simulink model "Test"  (R2018b)
settings: Solver=VariableStepAuto  StartTime=0.0  StopTime=10.0  RelTol=1e-3
undefined symbols (not defined in the file or in its folder): ExpectedOutputs, Inputs, sigbuilder_block, TestCase, TestInps, TestIters
libraries: fillib x3, library x2
(part 7 of 7)

== stateflow chart Test/Test Assessment Block2 ==
  settings: stateMachineType=SIMPLIFIED_MACHINE
  state Run
    if TestCase == 1
    verify(task_done ==  0);
    verify(inst_ptr == 0);
    verify(task_error == 0);
    verify(latch_addr ==  0)
    verify(write == 0)
    verify(ctrl == 0)
    verify(abort == 0)
    verify(fb_select == 0);
    end
    settings: description=|
        | Verify if in Init state all the outputs are reset to 0.
        | The instruction pointer should be reset to 0 to point to the first instruction in the sequence.
  state step2
    if TestCase == 2
    verify(task_done ==  0);
    verify(inst_ptr == 0);
    verify(task_error == 0);
    verify(latch_addr ==  0)
    verify(write == 0)
    verify(ctrl == 0)
    verify(abort == 0)
    verify(fb_select == 42);
    end
    settings: description=|
        | Verify that with a trigger from global sequencer, the task execution is initiated.
        | The state transitions from INIT to FB_SELECT.
        | Verify that the function number register and start instruction pointer register are latched to the first instruction in the sequence.
  state step3
    if TestCase == 2
    verify(task_done ==  0);
    verify(inst_ptr == 1);
    verify(task_error == 0);
    verify(latch_addr ==  0)
    verify(write == 0)
    verify(ctrl == 0)
    verify(abort == 0)
    verify(fb_select == 42);
    end
    settings: description=Verify that the instruction pointer increments.
  state step4
    if TestCase == 3
    verify(task_done ==  0);
    verify(inst_ptr == 1);
    verify(task_error == 0);
    verify(latch_addr ==  1)
    verify(int32(addr) == 32)
    verify(write == 0)
    verify(ctrl == 0)
    verify(abort == 0)
    verify(fb_select == 42);
    end
    settings: description=|
        | Verify that the state switches to Fetch automatically.
        | Verify that the fetch address in the instruction sequence is latched on the addr output.
  state step5
    if TestCase == 3
    verify(task_done ==  0);
    verify(inst_ptr == 1);
    verify(task_error == 0);
    verify(latch_addr ==  0)
    verify(write == 0)
    verify(ctrl == 0)
    verify(abort == 0)
    verify(fb_select == 42);
    end
    settings: description=Verify that there is one cycle of wait state for data to be available to function blocks from task memories.
  state step6
    if TestCase == 3
    verify(task_done ==  0);
    verify(inst_ptr == 1);
    verify(task_error == 0);
    verify(latch_addr ==  0)
    verify(write == 0)
    verify(ctrl == 1)
    verify(abort == 0)
    verify(fb_select == 42);
    end
    settings: description=Verify that a ctrl pulse is sent to function blocks to begin execution.
  state step7
    if TestCase == 3
    verify(task_done ==  0);
    verify(inst_ptr == 1);
    verify(task_error == 0);
    verify(latch_addr ==  0)
    verify(write == 0)
    verify(ctrl == 0)
    verify(abort == 0)
    verify(fb_select == 42);
    end
  state step8
    if TestCase == 3
    verify(task_done ==  0);
    verify(inst_ptr == 2);
    verify(task_error == 0);
    verify(latch_addr ==  0)
    verify(write == 0)
    verify(ctrl == 0)
    verify(abort == 0)
    verify(fb_select == 42);
    end
    settings: description=Verify that the instruction pointer is incremented.
  state step9
    if TestCase == 4
    verify(task_done ==  0);
    verify(inst_ptr == 2);
    verify(task_error == 0);
    verify(latch_addr ==  1)
    verify(write == 0)
    verify(ctrl == 0)
    verify(abort == 0)
    verify(fb_select == 42);
    end
    settings: description=|
        | Verify that the state remains in Fetch if the super state (upper 4 bits of Error Code in status signal) has not changed but the Error code data bits 22 through 27 has been incremented once indicating a super state iteration.
        | Verify that the next fetch address in the instruction sequence is latched on to the addr output.
  state step10
    if TestCase == 4
    verify(task_done ==  0);
    verify(inst_ptr == 2);
    verify(task_error == 0);
    verify(latch_addr ==  0)
    verify(write == 0)
    verify(ctrl == 0)
    verify(abort == 0)
    verify(fb_select == 42);
    end
    settings: description=Verify that there is one cycle of wait state for data to be available to function blocks from task memories.
  state step11
    if TestCase == 4
    verify(task_done ==  0);
    verify(inst_ptr == 2);
    verify(task_error == 0);
    verify(latch_addr ==  0)
    verify(write == 0)
    verify(ctrl == 1)
    verify(abort == 0)
    verify(fb_select == 42);
    end
    settings: description=Verify that a ctrl pulse is sent to function blocks to begin execution.
  state step12
    if TestCase == 4
    verify(task_done ==  0);
    verify(inst_ptr == 2);
    verify(task_error == 0);
    verify(latch_addr ==  0)
    verify(write == 0)
    verify(ctrl == 0)
    verify(abort == 0)
    verify(fb_select == 42);
    end
  state step13
    if TestCase == 4
    verify(task_done ==  0);
    verify(inst_ptr == 2);
    verify(task_error == 0);
    verify(latch_addr ==  0)
    verify(write == 0)
    verify(ctrl == 0)
    verify(abort == 0)
    verify(fb_select == 42);
    end
  state step14
    if TestCase == 4
    verify(task_done ==  0);
    verify(inst_ptr == 3);
    verify(task_error == 0);
    verify(latch_addr ==  0)
    verify(write == 0)
    verify(ctrl == 0)
    verify(abort == 0)
    verify(fb_select == 42);
    end
    settings: description=Verify that the instruction pointer is incremented.
  state step15
    if TestCase == 5
    verify(task_done ==  0);
    verify(inst_ptr == 3);
    verify(task_error == 0);
    verify(latch_addr ==  1)
    verify(write == 0)
    verify(ctrl == 0)
    verify(abort == 0)
    verify(fb_select == 42);
    end
    settings: description=|
        | Verify that the state remains in Fetch if the super state (upper 4 bits of Error Code in status signal) has not changed but the Error code data bits 22 through 27 has been incremented once indicating a super state iteration.
        | Verify that the next fetch address in the instruction sequence is latched on to the addr output.
  state step16
    if TestCase == 5
    verify(task_done ==  0);
    verify(inst_ptr == 3);
    verify(task_error == 0);
    verify(latch_addr ==  0)
    verify(write == 0)
    verify(ctrl == 0)
    verify(abort == 0)
    verify(fb_select == 42);
    end
    settings: description=Verify that there is one cycle of wait state for data to be available to function blocks from task memories.
  state step17
    if TestCase == 5
    verify(task_done ==  0);
    verify(inst_ptr == 3);
    verify(task_error == 0);
    verify(latch_addr ==  0)
    verify(write == 0)
    verify(ctrl == 1)
    verify(abort == 0)
    verify(fb_select == 42);
    end
    settings: description=Verify that a ctrl pulse is sent to function blocks.
  state step18
    if TestCase == 5
    verify(task_done ==  0);
    verify(inst_ptr == 3);
    verify(task_error == 0);
    verify(latch_addr ==  0)
    verify(write == 0)
    verify(ctrl == 0)
    verify(abort == 0)
    verify(fb_select == 42);
    end
  state step19
    if TestCase == 5
    verify(task_done ==  0);
    verify(inst_ptr == 3);
    verify(task_error == 0);
    verify(latch_addr ==  0)
    verify(write == 0)
    verify(ctrl == 0)
    verify(abort == 0)
    verify(fb_select == 42);
    end
  state step20
    if TestCase == 5
    verify(task_done ==  0);
    verify(inst_ptr == 4);
    verify(task_error == 0);
    verify(latch_addr ==  0)
    verify(write == 0)
    verify(ctrl == 0)
    verify(abort == 0)
    verify(fb_select == 42);
    end
    settings: description=Verify that the instruction pointer is incremented.
  state step21
    if TestCase == 6
    verify(task_done ==  0);
    verify(inst_ptr == 4);
    verify(task_error == 0);
    verify(latch_addr ==  0)
    verify(write == 0)
    verify(ctrl == 1)
    verify(abort == 0)
    verify(fb_select == 42);
    end
    settings: description=|
        | Verify that the state changes to Execute if the super state (upper 4 bits of Error Code in status signal) has changed indicating next state.
        | Verify that a ctrl pulse is sent to the function blocks for execution.
  state step22
    if TestCase == 6
    verify(task_done ==  0);
    verify(inst_ptr == 4);
    verify(task_error == 0);
    verify(latch_addr ==  0)
    verify(write == 0)
    verify(ctrl == 0)
    verify(abort == 0)
    verify(fb_select == 42);
    end
  state step23
    if TestCase == 7
    verify(task_done ==  0);
    verify(inst_ptr == 4);
    verify(task_error == 0);
    verify(latch_addr ==  1);
    verify(write == 0)
    verify(ctrl == 0)
    verify(abort == 0)
    verify(fb_select == 42);
    end
    settings: description=|
        | Verify that the state changes to Write if the super state (upper 4 bits of Error Code in status signal) has changed indicating next state.
        | Verify that the output address in the instruction sequence is latched on to the addr output.
  state step24
    if TestCase == 7
    verify(task_done ==  0);
    verify(inst_ptr == 4);
    verify(task_error == 0);
    verify(latch_addr ==  0);
    verify(write == 0)
    verify(ctrl == 1)
    verify(abort == 0)
    verify(fb_select == 42);
    end
    settings: description=Verify that a ctrl pulse is sent to function blocks.
  state step25
    if TestCase == 8
    verify(task_done ==  0);
    verify(inst_ptr == 4);
    verify(task_error == 0);
    verify(latch_addr ==  0);
    verify(write == 0)
    verify(ctrl == 0)
    verify(abort == 0)
    verify(fb_select == 42);
    end
  state step26
    if TestCase == 8
    verify(task_done ==  0);
    verify(inst_ptr == 4);
    verify(task_error == 0);
    verify(latch_addr ==  0);
    verify(write == 1)
    verify(ctrl == 0)
    verify(abort == 0)
    verify(fb_select == 42);
    end
    settings: description=Verify that the write output is set high to allow the function block to write the result to the current address.
  state step27
    if TestCase == 8
    verify(task_done ==  0);
    verify(inst_ptr == 4);
    verify(task_error == 0);
    verify(latch_addr ==  0);
    verify(write == 0)
    verify(ctrl == 0)
    verify(abort == 0)
    verify(fb_select == 42);
    end
  state step28
    if TestCase == 8
    verify(task_done ==  0);
    verify(inst_ptr == 5);
    verify(task_error == 0);
    verify(latch_addr ==  0);
    verify(write == 0)
    verify(ctrl == 0)
    verify(abort == 0)
    verify(fb_select == 42);
    end
    settings: description=Verify that the instruction pointer is incremented.
  state step29
    if TestCase == 9
    verify(task_done ==  0);
    verify(inst_ptr == 5);
    verify(task_error == 0);
    verify(latch_addr ==  1);
    verify(write == 0)
    verify(ctrl == 0)
    verify(abort == 0)
    verify(fb_select == 42);
    end
    settings: description=|
        | Verify that the state remains in Write if the super state (upper 4 bits of Error Code in status signal) has not changed but the Error code data bits 22 through 27 has been incremented once indicating a super state iteration.
        | Verify that the 2nd output address in the instruction sequence is latched on to the addr output.
  state step30
    if TestCase == 9
    verify(task_done ==  0);
    verify(inst_ptr == 5);
    verify(task_error == 0);
    verify(latch_addr ==  0);
    verify(write == 0)
    verify(ctrl == 1)
    verify(abort == 0)
    verify(fb_select == 42);
    end
    settings: description=Verify that a ctrl pulse is sent to function blocks.
  state step31
    if TestCase == 9
    verify(task_done ==  0);
    verify(inst_ptr == 5);
    verify(task_error == 0);
    verify(latch_addr ==  0);
    verify(write == 0)
    verify(ctrl == 0)
    verify(abort == 0)
    verify(fb_select == 42);
    end
  state step32
    if TestCase == 9
    verify(task_done ==  0);
    verify(inst_ptr == 5);
    verify(task_error == 0);
    verify(latch_addr ==  0);
    verify(write == 1)
    verify(ctrl == 0)
    verify(abort == 0)
    verify(fb_select == 42);
    end
    settings: description=Verify that the write output is set high to allow the function block to write the result to the current address.
  state step33
    if TestCase == 9
    verify(task_done ==  0);
    verify(inst_ptr == 5);
    verify(task_error == 0);
    verify(latch_addr ==  0);
    verify(write == 0)
    verify(ctrl == 0)
    verify(abort == 0)
    verify(fb_select == 42);
    end
  state step34
    if TestCase == 9
    verify(task_done ==  0);
    verify(inst_ptr == 6);
    verify(task_error == 0);
    verify(latch_addr ==  0);
    verify(write == 0)
    verify(ctrl == 0)
    verify(abort == 0)
    verify(fb_select == 42);
    end
    settings: description=Verify that the instruction pointer is incremented.
  state step35
    if TestCase == 9
    verify(task_done ==  0);
    verify(inst_ptr == 6);
    verify(task_error == 0);
    verify(latch_addr ==  0);
    verify(write == 0)
    verify(ctrl == 1)
    verify(abort == 0)
    verify(fb_select == 42);
    end
    settings: description=|
        | Verify that the state changes to FB_DONE if the super state (upper 4 bits of Error Code in status signal) has changed indicating next state.
        | Verify that a ctrl pulse is sent to function blocks to progress its state.
        | Verify that an Error while in FB_Done state does not cause it the local sequencer to move to the ERROR state.
  state step36
    if TestCase == 9
    verify(task_done ==  0);
    verify(inst_ptr == 6);
    verify(task_error == 0);
    verify(latch_addr ==  0);
    verify(write == 0)
    verify(ctrl == 0)
    verify(abort == 0)
    verify(fb_select == 42);
    end
  state step37
    if TestCase == 10
    verify(task_done ==  0);
    verify(inst_ptr == 6);
    verify(task_error == 0);
    verify(latch_addr ==  0);
    verify(write == 0)
    verify(ctrl == 0)
    verify(abort == 0)
    verify(fb_select == 42);
    end
    settings: description=Verify that the state changes to FB_SELECT if the super state (upper 4 bits of Error Code in status signal) has changed indicating next state.
  state step38
    if TestCase == 10
    verify(task_done ==  0);
    verify(inst_ptr == 6);
    verify(task_error == 0);
    verify(latch_addr ==  0);
    verify(write == 0)
    verify(ctrl == 0)
    verify(abort == 0)
    verify(fb_select == 41);
    end
    settings: description=Verify that the function number register and start instruction pointer register are latched to the 2nd function block instruction in the sequence.
  state step39
    if TestCase == 10
    verify(task_done ==  0);
    verify(inst_ptr == 7);
    verify(task_error == 0);
    verify(latch_addr ==  0);
    verify(write == 0)
    verify(ctrl == 0)
    verify(abort == 0)
    verify(fb_select == 41);
    end
    settings: description=|
        | Verify that the instruction pointer is incremented.
        | Verify that an Error while in FB_SELECT state does not cause it the local sequencer to move to the ERROR state.
  state step40
    if TestCase == 11
    verify(task_done ==  0);
    verify(inst_ptr == 7);
    verify(task_error == 0);
    verify(latch_addr ==  1);
    verify(write == 0)
    verify(ctrl == 0)
    verify(abort == 0)
    verify(fb_select == 41);
    end
    settings: description=|
        | Verify that the state switches to Fetch automatically.
        | Verify that the fetch address in the instruction sequence is latched on the addr output.
  state step41
    if TestCase == 11
    verify(task_done ==  0);
    verify(inst_ptr == 7);
    verify(task_error == 0);
    verify(latch_addr == 0);
    verify(write == 0)
    verify(ctrl == 1)
    verify(abort == 0)
    verify(fb_select == 41);
    end
    settings: description=|
        | Verify that the state switches to ERROR if the Error signal in Status input is true.
        | Verify that a ctrl pulse is sent to function blocks.
        | Verify that abort and Task_Error output signals are set to false if the lower 22 bits of the Code in Status signal indicate a recoverable error.
  state step42
    if TestCase == 11
    verify(task_done ==  0);
    verify(inst_ptr == 7);
    verify(task_error == 0);
    verify(latch_addr == 0);
    verify(write == 0)
    verify(ctrl == 0)
    verify(abort == 0)
    verify(fb_select == 41);
    end
  state step43
    if TestCase == 12
    verify(task_done ==  0);
    verify(inst_ptr == 7);
    verify(task_error == 0);
    verify(latch_addr == 0);
    verify(write == 0)
    verify(ctrl == 0)
    verify(abort == 0)
    verify(fb_select == 41);
    end
    settings: description=|
        | If the lower 22 bits of the Code in Status signal indicate a recoverable error,
        | verify that the state changes from ERROR to FB_SELECT.
  state step44
    if TestCase == 12
    verify(task_done ==  0);
    verify(inst_ptr == 6);
    verify(task_error == 0);
    verify(latch_addr == 0);
    verify(write == 0)
    verify(ctrl == 0)
    verify(abort == 0)
    verify(fb_select == 41);
    end
    settings: description=With a recoverable error verify that the instruction pointer is loaded with the value stored in the start instruction pointer register.
  state step45
    if TestCase == 12
    verify(task_done ==  0);
    verify(inst_ptr == 7);
    verify(task_error == 0);
    verify(latch_addr == 0);
    verify(write == 0)
    verify(ctrl == 0)
    verify(abort == 0)
    verify(fb_select == 41);
    end
    settings: description=Verify that the instruction pointer is incremented.
  state step46
    if TestCase == 13
    verify(task_done ==  0);
    verify(inst_ptr == 7);
    verify(task_error == 0);
    verify(latch_addr == 1);
    verify(write == 0)
    verify(ctrl == 0)
    verify(abort == 0)
    verify(fb_select == 41);
    end
    settings: description=|
        | Verify that the state switches to Fetch automatically.
        | Verify that the fetch address in the instruction sequence is latched on the addr output.
        | Verify that there is one cycle of wait state for data to be available to function blocks from task memories.
        | Verify that in the next cycle a ctrl pulse is sent to function blocks to begin execution.
        | Verify that after 2 cycles the instruction pointer is incremented.
  state step47
    if TestCase == 13
    verify(task_done ==  0);
    verify(inst_ptr == 7);
    verify(task_error == 0);
    verify(latch_addr == 0);
    verify(write == 0)
    verify(ctrl == 0)
    verify(abort == 0)
    verify(fb_select == 41);
    end
  state step48
    if TestCase == 13
    verify(task_done ==  0);
    verify(inst_ptr == 7);
    verify(task_error == 0);
    verify(latch_addr == 0);
    verify(write == 0)
    verify(ctrl == 1)
    verify(abort == 0)
    verify(fb_select == 41);
    end
  state step49
    if TestCase == 13
    verify(task_done ==  0);
    verify(inst_ptr == 7);
    verify(task_error == 0);
    verify(latch_addr == 0);
    verify(write == 0)
    verify(ctrl == 0)
    verify(abort == 0)
    verify(fb_select == 41);
    end
  state step50
    if TestCase == 13
    verify(task_done ==  0);
    verify(inst_ptr ==8)
    verify(task_error == 0);
    verify(latch_addr == 0)
    verify(write == 0)
    verify(ctrl == 0)
    verify(abort == 0)
    verify(fb_select == 41);
    end
  state step51
    if (TestCase == 14)
    verify(task_done ==  0);
    verify(inst_ptr ==8)
    verify(task_error == 0);
    verify(latch_addr == 0)
    verify(write == 0)
    verify(ctrl == 1)
    verify(abort == 0)
    verify(fb_select == 41);
    end
    settings: description=|
        | Verify that the state changes to Execute if the super state (upper 4 bits of Error Code in status signal) has changed indicating next state.
        | Verify that a ctrl pulse is sent to the function blocks for execution.
  state step52
    if (TestCase == 14)
    verify(task_done ==  0);
    verify(inst_ptr == 8)
    verify(task_error == 1);
    verify(latch_addr == 0)
    verify(write == 0)
    verify(ctrl == 1)
    verify(abort == 1)
    verify(fb_select == 41);
    end
    settings: description=|
        | Verify that the state switches to ERROR if the Error signal in Status input is true.
        | If the lower 22 bits of the Code in Status signal indicate a non recoverable error, verify that a ctrl and abort signals are pulsed for one cycle.
        | Verify that the Task_Error output is set to true until the Trigger goes low.
  state step53
    if (TestCase == 14)
    verify(task_done ==  0);
    verify(inst_ptr == 8)
    verify(task_error == 1);
    verify(latch_addr == 0)
    verify(write == 0)
    verify(ctrl == 0)
    verify(abort == 0)
    verify(fb_select == 41);
    end
  state step54
    if (TestCase == 15)
    verify(task_done ==  0);
    verify(inst_ptr == 0)
    verify(task_error == 0);
    verify(latch_addr == 0)
    verify(write == 0)
    verify(ctrl == 0)
    verify(abort == 0)
    verify(fb_select == 0);
    end
    settings: description=|
        | Verify that the state transitions from ERROR state to INIT if the error is not recoverable and the trigger from the global sequencer is low.
        | Verify if in Init state all the outputs are reset to 0.
        | The instruction pointer should be reset to 0 to point to the first instruction in the sequence
  state step55
    if (TestCase == 16)
    verify(task_done ==  0);
    verify(inst_ptr == 0)
    verify(task_error == 0);
    verify(latch_addr == 0)
    verify(write == 0)
    verify(ctrl == 0)
    verify(abort == 0)
    verify(fb_select == 50);
    end
    settings: description=|
        | Verify that with a trigger from global sequencer, the task execution is initiated.
        | The state transitions from INIT to FB_SELECT.
        | Verify that the function number register and start instruction pointer register are latched to the first instruction in the sequence.
  state step_1
  state step56
    if TestCase == 16
    verify(task_done ==  0);
    verify(inst_ptr == 2)
    verify(task_error == 0);
    verify(latch_addr == 1)
    verify(write == 0)
    verify(ctrl == 0)
    verify(abort == 0)
    verify(fb_select == 50);
    end
    settings: description=Verify that the write state is entered.
  state step_57
    if TestCase == 16
    verify(task_done ==  0);
    verify(inst_ptr == 2)
    verify(task_error == 0);
    verify(latch_addr == 0)
    verify(write == 0)
    verify(ctrl == 1)
    verify(abort == 0)
    verify(fb_select == 50);
    end
    settings: description=Verify that Error state is entered from write state if error is detected.
  state step_58
    if TestCase == 16
    verify(task_done ==  0);
    verify(inst_ptr == 2)
    verify(task_error == 0);
    verify(latch_addr == 0)
    verify(write == 0)
    verify(ctrl == 0)
    verify(abort == 0)
    verify(fb_select == 50);
    end
  state step59
    if TestCase ==16
    verify(task_done ==  0);
    verify(inst_ptr == 0)
    verify(task_error == 0);
    verify(latch_addr == 0)
    verify(write == 0)
    verify(ctrl == 0)
    verify(abort == 0)
    verify(fb_select == 50);
    end
  state step60
  state step61
    if (TestCase == 17)
    verify(task_done ==  1);
    verify(inst_ptr == 3)
    verify(task_error == 0);
    verify(latch_addr == 0)
    verify(write == 0)
    verify(ctrl == 0)
    verify(abort == 0)
    verify(fb_select == 50);
    end
    settings: description=Verify that state moves to Task_Done from FB_Done state once function block signals a new state and EOF flag is the current instruction.
  state step63
    if (TestCase == 18)
    verify(task_done ==  0);
    verify(inst_ptr == 3)
    verify(task_error == 0);
    verify(latch_addr == 0)
    verify(write == 0)
    verify(ctrl == 0)
    verify(abort == 0)
    verify(fb_select == 50);
    end
    settings: description=Verify that the state moves from Task_Done to INIT state once Trigger goes low.
  state step64
    if (TestCase == 18)
    verify(task_done ==  0);
    verify(inst_ptr == 0)
    verify(task_error == 0);
    verify(latch_addr == 0)
    verify(write == 0)
    verify(ctrl == 0)
    verify(abort == 0)
    verify(fb_select == 0);
    end
  state step65
  state step66
    if ((TestCase == 19)||(TestCase == 20)||(TestCase == 21)||(TestCase == 22))
    verify(task_done ==  0);
    verify(inst_ptr == 1)
    verify(task_error == 1);
    verify(latch_addr == 0)
    verify(write == 0)
    verify(ctrl == 1)
    verify(abort == 1)
    verify(fb_select == 52);
    elseif((TestCase == 23)||(TestCase == 24)||(TestCase == 25)||(TestCase == 26)||(TestCase == 27)||(TestCase == 28) || (TestCase == 29) ||  (TestCase == 30))
    verify(task_done ==  0);
    verify(inst_ptr == 2)
    verify(task_error == 1);
    verify(latch_addr == 0)
    verify(write == 0)
    verify(ctrl == 1)
    verify(abort == 1)
    verify(fb_select == 52);
    elseif((TestCase == 31) || (TestCase == 32))
    verify(task_done ==  0);
    verify(inst_ptr == 3)
    verify(task_error == 1);
    verify(latch_addr == 0)
    verify(write == 0)
    verify(ctrl == 1)
    verify(abort == 1)
    verify(fb_select == 52);
    end
  state EndTest
  (default) -> Run
  Run -> (junction 371) [order 2] : [after(3,sec) && (TestCase == 1)
      | ]
  (junction 371) -> (junction 363)
  Run -> step2 [order 1] : [after(3,sec) && TestCase > 1
      | ]
  step2 -> step3 : [after(1,sec)
      | ]
  step3 -> (junction 363) [order 2] : [after(1,sec) && TestCase == 2
      | ]
  (junction 363) -> (junction 304)
  step3 -> step4 [order 1] : [after(1,sec) && TestCase > 2
      | ]
  step4 -> step5 : [after(1,sec)
      | ]
  step5 -> step6 : [after(1,sec)
      | ]
  step6 -> step7 : [after(1,sec)
      | ]
  step7 -> step8 : [after(2, sec)
      | ]
  step8 -> (junction 304) [order 2] : [after(1,sec) && TestCase == 3
      | ]
  (junction 304) -> (junction 307)
  step8 -> step9 [order 1] : [after(1,sec) && TestCase > 3
      | ]
  step9 -> step10 : [after(1,sec)
      | ]
  step10 -> step11 : [after(1,sec)
      | ]
  step11 -> step12 : [after(1,sec)
      | ]
  step12 -> step13 : [after(1,sec)
      | ]
  step13 -> step14 : [after(1,sec)
      | ]
  step14 -> (junction 307) [order 2] : [after(1,sec) && TestCase == 4
      | ]
  (junction 307) -> (junction 310)
  step14 -> step15 [order 1] : [after(1,sec) && TestCase > 4
      | ]
  step15 -> step16 : [after(1,sec)
      | ]
  step16 -> step17 : [after(1,sec)
      | ]
  step17 -> step18 : [after(1,sec)
      | ]
  step18 -> step19 : [after(1,sec)
      | ]
  step19 -> step20 : [after(1,sec)
      | ]
  step20 -> (junction 310) [order 2] : [after(3,sec) && TestCase == 5
      | ]
  (junction 310) -> (junction 313)
  step20 -> step21 [order 1] : [after(3,sec) && TestCase > 5
      | ]
  step21 -> step22 : [after(1,sec)
      | ]
  step22 -> (junction 313) [order 2] : [after(1,sec) && TestCase == 6
      | ]
  (junction 313) -> (junction 320)
  step22 -> step23 [order 1] : [after(1,sec) && TestCase > 6
      | ]
  step23 -> step24 : [after(1,sec)
      | ]
  step24 -> step25 : [after(1,sec)
      | ]
  step25 -> step26 : [after(1,sec)
      | ]
  step26 -> step27 : [after(1,sec)
      | ]
  step27 -> step28 : [after(1,sec)
      | ]
  step28 -> (junction 320) [order 2] : [after(2,sec) && TestCase == 7
      | ]
  (junction 320) -> (junction 323)
  step28 -> step29 [order 1] : [after(2,sec) && TestCase > 7
      | ]
  step29 -> step30 : [after(1,sec)
      | ]
  step30 -> step31 : [after(1,sec)
      | ]
  step31 -> step32 : [after(1,sec)
      | ]
  step32 -> step33 : [after(1,sec)
      | ]
  step33 -> step34 : [after(1,sec)
      | ]
  step34 -> (junction 323) [order 2] : [after(1,sec) && TestCase == 8
      | ]
  (junction 323) -> (junction 326)
  step34 -> step35 [order 1] : [after(1,sec) && TestCase > 8
      | ]
  step35 -> step36 : [after(1,sec)
      | ]
  step36 -> (junction 326) [order 2] : [after(1,sec) && TestCase == 9
      | ]
  (junction 326) -> (junction 329)
  step36 -> step37 [order 1] : [after(1,sec) && TestCase > 9
      | ]
  step37 -> step38 : [after(2,sec)
      | ]
  step38 -> step39 : [after(1,sec)
      | ]
  step39 -> (junction 329) [order 2] : [after(1,sec) && TestCase == 10
      | ]
  (junction 329) -> (junction 332)
  step39 -> step40 [order 1] : [after(1,sec) && TestCase > 10
      | ]
  step40 -> step41 : [after(1,sec)
      | ]
  step41 -> step42 : [after(1,sec)
      | ]
  step42 -> (junction 332) [order 2] : [after(1,sec) && TestCase == 11
      | ]
  (junction 332) -> (junction 335)
  step42 -> step43 [order 1] : [after(1,sec) && TestCase > 11
      | ]
  step43 -> step44 : [after(1,sec)
      | ]
  step44 -> step45 : [after(1,sec)
      | ]
  step45 -> (junction 335) [order 2] : [after(1,sec) && TestCase == 12
      | ]
  (junction 335) -> (junction 338)
  step45 -> step46 [order 1] : [after(1,sec) && TestCase > 12
      | ]
  step46 -> step47 : [after(1,sec)
      | ]
  step47 -> step48 : [after(1,sec)
      | ]
  step48 -> step49 : [after(1,sec)
      | ]
  step49 -> step50 : [after(2,sec)
      | ]
  step50 -> (junction 338) [order 2] : [after(3,sec) && TestCase == 13
      | ]
  (junction 338) -> (junction 539)
  step50 -> step51 [order 1] : [after(3,sec) && TestCase > 13
      | ]
  step51 -> step52 : [after(1,sec)
      | ]
  step52 -> step53 : [after(1,sec)
      | ]
  step53 -> (junction 539) [order 2] : [after(5,sec) && (TestCase == 14)
      | ]
  (junction 539) -> (junction 344)
  step53 -> step54 [order 1] : [after(5,sec) && TestCase > 14
      | ]
  step54 -> (junction 344) [order 2] : [after(3,sec) && TestCase == 15
      | ]
  (junction 344) -> (junction 496)
  step54 -> step55 [order 1] : [after(3,sec) && TestCase > 15
      | ]
  step55 -> step_1 : [after(1,sec)
      | ]
  step_1 -> step56 : [after(13,sec)
      | ]
  step56 -> step_57 : [after(1,sec)
      | ]
  step_57 -> step_58 : [after(1,sec)
      | ]
  step_58 -> step59 : [after(2,sec)
      | ]
  step59 -> (junction 496) [order 1] : [after(1,sec) && TestCase == 16
      | ]
  (junction 496) -> (junction 510)
  step59 -> step60 [order 2] : [after(1,sec) && TestCase> 16
      | ]
  step60 -> step61 : [after(27,sec)
      | ]
  step61 -> (junction 510) [order 1] : [after(2,sec) && TestCase == 17
      | ]
  (junction 510) -> (junction 543)
  step61 -> step63 [order 2] : [after(2,sec) && TestCase > 17
      | ]
  step63 -> step64 : [after(1,sec)
      | ]
  step64 -> (junction 543) [order 1] : [after(1, sec) && TestCase == 18
      | ]
  (junction 543) -> (junction 295)
  step64 -> step65 [order 2] : [after(1,sec) && TestCase > 18
      | ]
  step65 -> step66 [order 7] : [after(9,sec) && TestCase == 25
      | ]
  step65 -> step66 [order 8] : [after(10,sec) && TestCase == 26
      | ]
  step65 -> step66 [order 9] : [after(11,sec) && TestCase == 27
      | ]
  step65 -> step66 [order 10] : [after(12,sec) && TestCase == 28
      | ]
  step65 -> step66 [order 11] : [after(13,sec) && TestCase == 29
      | ]
  step65 -> step66 [order 12] : [after(14,sec) && TestCase == 30
      | ]
  step65 -> step66 [order 13] : [after(15,sec) && TestCase == 31
      | ]
  step65 -> step66 [order 1] : [after(3,sec) && TestCase == 19
      | ]
  step65 -> step66 [order 2] : [after(4,sec) && TestCase == 20
      | ]
  step65 -> step66 [order 3] : [after(5,sec) && TestCase == 21
      | ]
  step65 -> step66 [order 4] : [after(6,sec) && TestCase == 22
      | ]
  step65 -> step66 [order 5] : [after(7,sec) && TestCase == 23
      | ]
  step65 -> step66 [order 6] : [after(8,sec) && TestCase == 24
      | ]
  step65 -> step66 [order 14] : [after(16,sec) && TestCase == 32
      | ]
  step66 -> EndTest
  (junction 295) -> EndTest
  data: task_error input boolean size=[1]; task_done input boolean size=[1]; inst_ptr input uint32 size=[1]; addr input; write input boolean size=[1]; ctrl input boolean size=[1]; abort input boolean size=[1]; fb_select input uint8 size=[1]; latch_addr input boolean size=[1]; TestCase parameter

== stateflow chart Test/Test Sequence7 ==
  settings: stateMachineType=SIMPLIFIED_MACHINE
  state Run
    %% Initialize data outputs.
    trigger = false;
    inst = 42;
    status.done = false;
    status.busy = false;
    status.error = false;
    status.code = uint32(0);
    settings: description=Init State
  state step_1
    trigger = true;
    settings: description=Trigger from Global Sequencer made True
  state step_2
    inst = 42;
    settings: description=|
        | Set inst to 42 indicating a function block corresponding to the enumeration
        | 42 to be selected by the Local sequencer
  state step_3
    inst = 32;
    status.code = uint32(0);
    settings: description=|
        | Set the next instruction to 32. This becomes the 8bit memory adress for fetching
        |  the first input for the function block
  state step_4
    status.code = uint32(4194304);
    settings: description=|
        | Set the code bits of the code such that the 22-27 bits increment by 1 indicating
        | a 2nd input to fetch.
  state step_5
    status.code = uint32(8388608);
    settings: description=|
        | Set the code bits of the code such that the 22-27 bits again increments by 1 indicating
        | a 3rd input to fetch.
  state step_6
    status.code = uint32(268435456)
    settings: description=|
        | Set the code bits such that the upper 4 bits change from the previous value indicating
        |  Local Sequencer to transition to the Execute.
  state step_7
    status.code = uint32(536870912)
    settings: description=|
        | Set the code bits such that the uppr four bits change value from previous value
        |  indicating Local sequencer to transition to the Write output state
  state step_8
    status.code = uint32(541065216)
    inst = 41
    settings: description=|
        | Set the code bits of the code such that the 22-27 bits increments by 1 indicating
        | a 2nd input to fetch.
  state step_9
    status.code = uint32(805306369)
    settings: description=|
        | Set the code bits such that the uppr four bits change value from previous value
        |  indicating Local sequencer to transition to the FB Done state.
  state step_10
    status.error = logical(1);
    settings: description=Check that error while in FB_Done and FB_select sate will be ignored.
  state step_11
    status.code = uint32(0)
  state step_12
    status.code = uint32(4194305)
    settings: description=Set the error as Recoverable.
  state step_13
    status.error = logical(0);
  state step_14
    status.code = uint32(268435456);
  state step_15
    status.error = logical(1);
  state step_16
    trigger =false;
    inst = 42;
    status.error = logical(0);
  state step_17
    trigger = true;
    status.code = uint32(0);
    inst =50;
    settings: description=Verify that a recoverable Error in Write state causes it to move to the Error state and further to the FBSelect state.
  state step_18
    status.code = uint32(268435456);
  state step_19
    status.code = uint32(536870912);
  state step_20
    status.error = logical(1);
    status.code = uint32(4194305)
  state step_21
    status.error = logical(0);
    status.code = uint32(0);
    inst =50;
    settings: description=Read FB_Select state
  state step_22
    status.code = uint32(268435456);
    settings: description=Reach Fetch state
  state step_23
    status.code = uint32(536870912)
    settings: description=Reach Execute state
  state step_24
    status.code = uint32(805306369)
    settings: description=Reach Write state
  state step_25
    status.code = uint32(1073741824)
    settings: description=Reach FB_Done state
  state step_26
    status.code = uint32(1342177280)
    inst = 2147483647
    settings: description=Reach Task Done state due to EOF.
  state step_27
    trigger = false;
  state step_28
    trigger = true;
    inst=52;
    status.code = uint32(0);
  state step_29
  state step_30
    status.code = uint32(268435456);
    settings: description=Verify that Error state is entered from all of the substates of Fetch state if Error is detected.
  state step_31
    status.code = uint32(536870912)
    settings: description=Verify that Error state is entered from all of the substates of Write state if Error is detected.
  state step_32
    status.error = logical(1);
  state EndTest
  (junction 368) -> (junction 370)
  (default) -> Run
  Run -> (junction 99) [order 2] : [after(1,sec) && TestCase == 1
      | ]
  (junction 99) -> (junction 103)
  Run -> step_1 [order 1] : [after(1,sec) && TestCase >1
      | ]
  step_1 -> step_2 : [after(1,sec)
      | ]
  step_2 -> (junction 103) [order 2] : [after(1,sec) && TestCase == 2
      | ]
  (junction 103) -> (junction 106)
  step_2 -> step_3 [order 1] : [after(1,sec) && TestCase > 2
      | ]
  step_3 -> (junction 106) [order 2] : [after(7,sec) && TestCase == 3
      | ]
  (junction 106) -> (junction 109)
  step_3 -> step_4 [order 1] : [after(7,sec) && TestCase > 3
      | ]
  step_4 -> (junction 109) [order 2] : [after(6,sec) && TestCase == 4
      | ]
  (junction 109) -> (junction 112)
  step_4 -> step_5 [order 1] : [after(6,sec) && TestCase > 4
      | ]
  step_5 -> (junction 112) [order 2] : [after(8,sec) && TestCase == 5
      | ]
  (junction 112) -> (junction 115)
  step_5 -> step_6 [order 1] : [after(8,sec) && TestCase > 5
      | ]
  step_6 -> (junction 115) [order 2] : [after(2,sec) && TestCase == 6
      | ]
  (junction 115) -> (junction 118)
  step_6 -> step_7 [order 1] : [after(2,sec) && TestCase > 6
      | ]
  step_7 -> (junction 118) [order 2] : [after(7,sec) && TestCase == 7
      | ]
  (junction 118) -> (junction 122)
  step_7 -> step_8 [order 1] : [after(7,sec) && TestCase > 7
      | ]
  step_8 -> (junction 122) [order 2] : [after(6,sec) && TestCase == 8
      | ]
  (junction 122) -> (junction 124)
  step_8 -> step_9 [order 1] : [after(6,sec) && TestCase > 8
      | ]
  step_9 -> (junction 124) [order 2] : [after(2,sec) && TestCase == 9
      | ]
  (junction 124) -> (junction 133)
  step_9 -> step_10 [order 1] : [after(2,sec) && TestCase > 9
      | ]
  step_10 -> step_11 : [after(1,sec)
      | ]
  step_11 -> (junction 133) [order 2] : [after(4,sec) && TestCase == 10
      | ]
  (junction 133) -> (junction 129)
  step_11 -> step_12 [order 1] : [after(4,sec) && TestCase > 10
      | ]
  step_12 -> (junction 129) [order 2] : [after(6,sec) && TestCase == 11
      | ]
  (junction 129) -> (junction 138)
  step_12 -> step_13 [order 1] : [after(6,sec) && TestCase > 11
      | ]
  step_13 -> (junction 138) [order 2] : [after(7,sec) && TestCase == 12
      | ]
  (junction 138) -> (junction 141)
  step_13 -> step_14 [order 1] : [after(7,sec) && TestCase > 12
      | ]
  step_14 -> step_15 : [after(1,sec)
      | ]
  step_15 -> (junction 141) [order 2] : [after(5,sec) && TestCase == 14
      | ]
  (junction 141) -> (junction 144)
  step_15 -> step_16 [order 1] : [after(5,sec) && TestCase > 14
      | ]
  step_16 -> (junction 144) [order 2] : [after(3,sec) && TestCase == 15
      | ]
  (junction 144) -> (junction 241)
  step_16 -> step_17 [order 1] : [after(3,sec) && TestCase > 15
      | ]
  step_17 -> step_18 : [after(9,sec)
      | ]
  step_18 -> step_19 : [after(6,sec)
      | ]
  step_19 -> step_20 : [after(1,sec)
      | ]
  step_20 -> step_21 : [after(4,sec)
      | ]
  step_21 -> (junction 241) [order 1] : [after(6,sec) && TestCase == 16
      |
      | ]
  (junction 241) -> (junction 247)
  step_21 -> step_22 [order 2] : [after(6,sec) && TestCase > 16
      | ]
  step_22 -> step_23 : [after(6,sec)
      | ]
  step_23 -> step_24 : [after(6,sec)
      | ]
  step_24 -> step_25 : [after(6,sec)
      | ]
  step_25 -> step_26 : [after(3,sec)
      | ]
  step_26 -> (junction 247) [order 1] : [after(2,sec) && TestCase == 17
      | ]
  (junction 247) -> (junction 254)
  step_26 -> step_27 [order 2] : [after(2,sec) && TestCase > 17
      | ]
  step_27 -> (junction 254) [order 1] : [after(1,sec) && TestCase == 18
      | ]
  (junction 254) -> (junction 97)
  step_27 -> step_28 [order 2] : [after(1,sec) && TestCase > 18
      | ]
  step_28 -> step_29 : [after(1,sec)
      | ]
  step_29 -> (junction 358) [order 1] : [after(3,sec) && TestCase == 19
      | ]
  (junction 358) -> (junction 360)
  step_29 -> (junction 360) [order 2] : [after(4,sec) && TestCase == 20
      | ]
  (junction 360) -> (junction 363)
  step_29 -> (junction 363) [order 3] : [after(5,sec) && TestCase == 21
      | ]
  (junction 363) -> (junction 365)
  step_29 -> (junction 368) [order 5] : [after(7,sec) && TestCase == 23
      | ]
  step_29 -> (junction 365) [order 4] : [after(6,sec) && TestCase == 22
      | ]
  (junction 365) -> (junction 368)
  step_29 -> (junction 370) [order 6] : [after(8,sec) && TestCase == 24
      | ]
  (junction 370) -> (junction 375)
  step_29 -> step_30 [order 7] : [after(8,sec) && TestCase > 24
      | ]
  step_30 -> (junction 375) [order 1] : [after(1,sec) && TestCase == 25
      | ]
  (junction 375) -> (junction 379)
  step_30 -> (junction 379) [order 2] : [after(2,sec) && TestCase == 26
      | ]
  (junction 379) -> (junction 288)
  step_30 -> step_31 [order 3] : [after(2,sec) && TestCase > 26
      | ]
  step_31 -> step_32 [order 1] : [after(1,sec) && TestCase == 27
      | ]
  step_31 -> step_32 [order 2] : [after(2,sec) && TestCase == 28
      | ]
  step_31 -> step_32 [order 3] : [after(3,sec) && TestCase == 29
      | ]
  step_31 -> step_32 [order 4] : [after(4,sec) && TestCase == 30
      | ]
  step_31 -> step_32 [order 5] : [after(5,sec) && TestCase == 31
      | ]
  step_31 -> step_32 [order 6] : [after(6,sec) && TestCase == 32
      | ]
  (junction 288) -> step_32
  step_32 -> EndTest
  (junction 97) -> EndTest
  data: trigger output boolean size=[1]; inst output int32 size=[1]; status output Bus: fb_status size=[1]; TestCase parameter uint8
